simulink model "ask"  (Simulink 7.4)
settings: Solver=ode45  StartTime=0.0  StopTime=10.0  RelTol=1e-3
libraries: commrandsrc2 x1, dspmathops x1
settings Model: Creator=divyata  LastModifiedBy=divyata

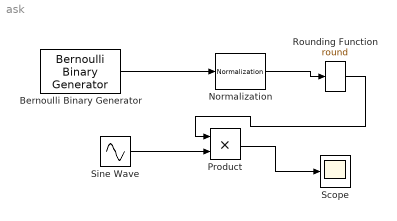
== system ask ==
  Bernoulli Binary Generator : commrandsrc2/Bernoulli Binary Generator  DialogController=commDDGCreate  DialogControllerArgs=DataTag0  SystemSampleTime=-1  P=0.5  seed=61  Ts=1  frameBased=off  sampPerFrame=1  orient=off  outDataType=double
  Normalization : dspmathops/Normalization  DialogController=dspDDGCreate  DialogControllerArgs=DataTag1  NormType=Squared 2-norm  Bias=1e-10  NormOver=Each column  ColComp=on  Dimension=1  outputDataTypeStr=Inherit: Same as product output  outputLastDataTypeStr=Inherit: Same as product output  outputMin=[]  outputMax=[]  accumDataTypeStr=Inherit: Same as product output  accumLastDataTypeStr=Inherit: Same as product output  roundingMode=Floor  overflowMode=off
  Product : Product  OutDataType=fixdt(1, 16)  OutScaling=2^0  RndMeth=Zero
  Rounding Function : Rounding  Operator=round
  Scope : Scope
  Sine Wave : Sin  Amplitude=1  Bias=0  Frequency=10000  Phase=pi./2  Samples=10  SampleTime=0  Offset=0
  wires:
  Bernoulli Binary Generator/1 -> Normalization/1
  Normalization/1 -> Rounding Function/1
  Sine Wave/1 -> Product/2
  Rounding Function/1 -> Product/1
  Product/1 -> Scope/1
